simulink model "mpc_test"  (R2023a)
settings: Solver=VariableStepAuto  StartTime=0.0  StopTime=500  RelTol=1e-3
libraries: cstblocks x2, mpclib x1
settings Model: Creator=Yuganshu Wadhwa  LastModifiedBy=Yuganshu Wadhwa

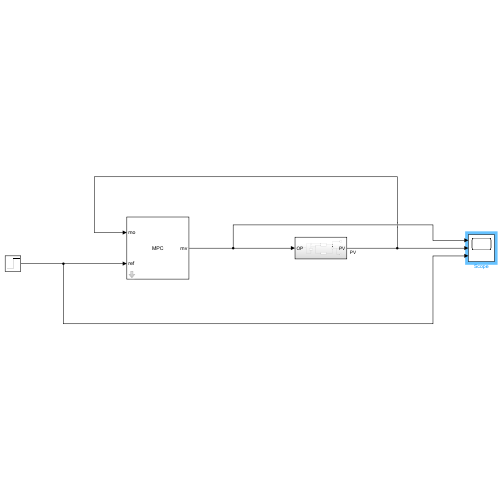
[thumbnail: Simulink's stored preview of the top-level diagram]
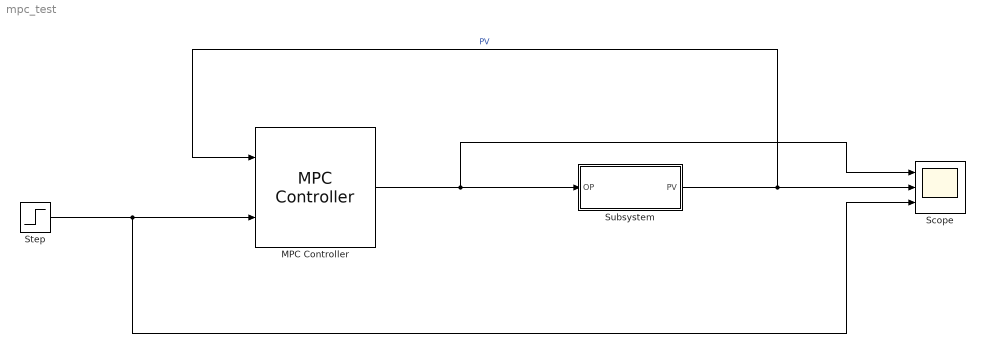
== system mpc_test ==
  MPC Controller : mpclib/MPC Controller  SCDEnableBlockLinearizationSpecification=on  mpcobj=mpc1  is_multiple=0  enable_value=0  return_u0=off  updateMPCinCallerWorkspace=on  md_inport=off  mv_inport=off  uref_inport=off  return_cost=off  return_mvseq=off  return_qpstatus=off  return_xseq=off  return_state=off  return_ovseq=off  state_inport=off  umin_inport=off  umax_inport=off  ymin_inport=off  ymax_inport=off  cc_inport=off  ywt_inport=off  uwt_inport=off  duwt_inport=off  rhoeps_inport=off  pm_inport=off  MaximumP=10  HorizonChoice=FixedHorizon  n_ts=1  n_p=30  n_mv=1  n_md=0  n_ud=0  n_mo=1  n_uo=0  BlockDataType=double  SampleTimeInherited=off  switch_inport=off
  Scope : Scope  NumInputPorts=3
  Step : Step  Time=200  Before=32  After=33  SampleTime=0
  Subsystem : Subsystem
  wires:
  MPC Controller/1 -> Scope/1, Subsystem/1(OP)
  Subsystem/1(PV) -> MPC Controller/1, Scope/2  "PV"
  Step/1 -> Scope/3, MPC Controller/2

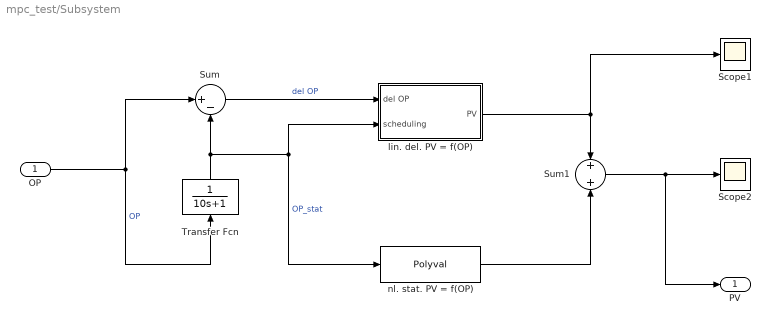
== system mpc_test/Subsystem ==
  OP : Inport
  Scope1 : Scope
  Scope2 : Scope
  Sum : Sum  Inputs=|+-
  Sum1 : Sum  Inputs=+|+
  Transfer Fcn : TransferFcn  Denominator=[10 1]
  "lin. del. PV = f(OP) " : Subsystem
  nl. stat. PV = f(OP) : Polyval  Coefs=[ -0.0004, +0.0693, +30.896 ]
  PV : Outport
  wires:
  nl. stat. PV = f(OP)/1 -> Sum1/2
  "lin. del. PV = f(OP) "/1(PV) -> Scope1/1, Sum1/1
  Sum1/1 -> Scope2/1, PV/1
  Sum/1 -> "lin. del. PV = f(OP) "/1(del OP)  "del OP"
  OP/1 -> Sum/1, Transfer Fcn/1  "OP"
  Transfer Fcn/1 -> nl. stat. PV = f(OP)/1, "lin. del. PV = f(OP) "/2(scheduling), Sum/2  "OP_stat"

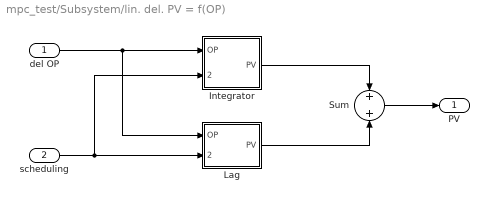
== system mpc_test/Subsystem/lin. del. PV = f(OP)  ==
  del OP : Inport
  scheduling : Inport  Port=2
  Integrator : Subsystem
  Lag : Subsystem
  Sum : Sum  Inputs=+|+
  PV : Outport
  wires:
  Lag/1(PV) -> Sum/2
  Sum/1 -> PV/1
  scheduling/1 -> Integrator/2(scheduling), Lag/2(scheduling)
  del OP/1 -> Lag/1(OP), Integrator/1(OP)
  Integrator/1(PV) -> Sum/1

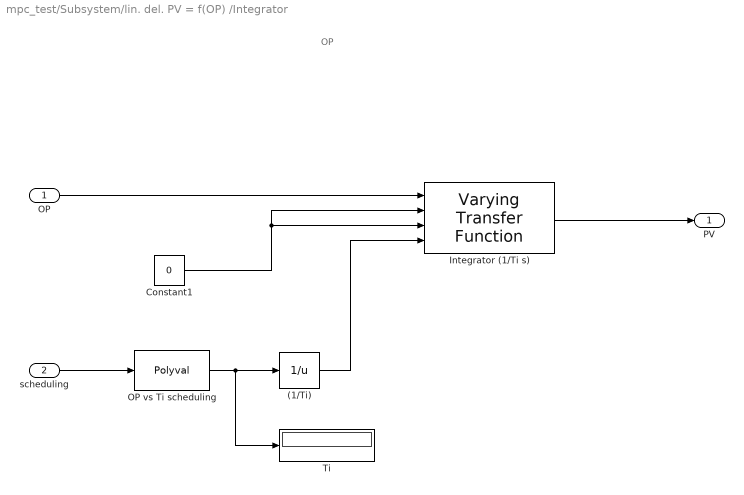
== system mpc_test/Subsystem/lin. del. PV = f(OP) /Integrator ==
  note: OP
  OP : Inport
  scheduling : Inport  Port=2
  (1/Ti) : Math  Operator=reciprocal
  Constant1 : Constant  Value=0
  Integrator (1/Ti s) : cstblocks/Linear Parameter Varying/Varying Transfer Function  N=1  Feedthrough=on
  OP vs Ti scheduling : Polyval  Coefs=[ +0.3812, -72.91, +4942.1, -110789, +1e+06 ]
  Ti : Display
  PV : Outport
  wires:
  OP/1 -> Integrator (1/Ti s)/1
  Constant1/1 -> Integrator (1/Ti s)/3, Integrator (1/Ti s)/2
  OP vs Ti scheduling/1 -> Ti/1, (1/Ti)/1
  Integrator (1/Ti s)/1 -> PV/1
  (1/Ti)/1 -> Integrator (1/Ti s)/4
  scheduling/1 -> OP vs Ti scheduling/1

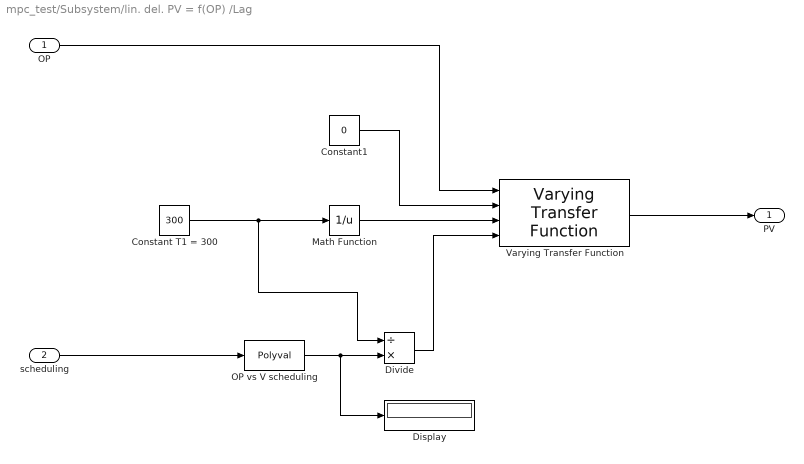
== system mpc_test/Subsystem/lin. del. PV = f(OP) /Lag ==
  OP : Inport
  scheduling : Inport  Port=2
  Constant T1 = 300 : Constant  Value=300
  Constant1 : Constant  Value=0
  Display : Display
  Divide : Product  Inputs=/*
  Math Function : Math  Operator=reciprocal
  OP vs V scheduling : Polyval  Coefs="[  -3e-7, +8e-5, -0.0065, 0.1944 ]"
  Varying Transfer Function : cstblocks/Linear Parameter Varying/Varying Transfer Function  N=1  Feedthrough=on
  PV : Outport
  wires:
  Divide/1 -> Varying Transfer Function/4
  Constant T1 = 300/1 -> Math Function/1, Divide/1
  Constant1/1 -> Varying Transfer Function/2
  OP/1 -> Varying Transfer Function/1
  OP vs V scheduling/1 -> Display/1, Divide/2
  Math Function/1 -> Varying Transfer Function/3
  Varying Transfer Function/1 -> PV/1
  scheduling/1 -> OP vs V scheduling/1
